simulink model "Model"  (Simulink 7.1)
settings: Solver=ode3  StartTime=0.0  StopTime=30.0  FixedStep=0.01  RelTol=1e-3
settings Model: Creator=Michal  LastModifiedBy=Michal

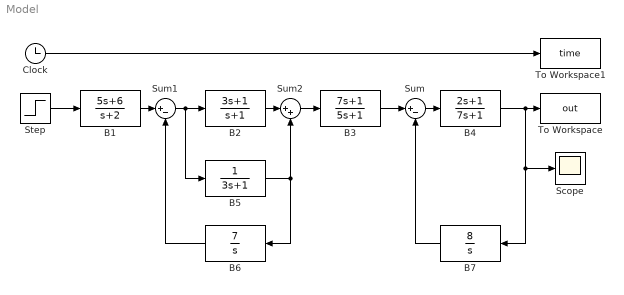
== system Model ==
  B1 : TransferFcn  Numerator=[5 6 ]  Denominator=[1 2]
  B2 : TransferFcn  Numerator=[3 1]  Denominator=[1 1]
  B3 : TransferFcn  Numerator=[7 1]  Denominator=[5 1]
  B4 : TransferFcn  Numerator=[2 1]  Denominator=[7 1]
  B5 : TransferFcn  Denominator=[3 1]
  B6 : TransferFcn  Orientation=left  Numerator=[7]  Denominator=[1 0]
  B7 : TransferFcn  Orientation=left  Numerator=[8]  Denominator=[1 0]
  Clock : Clock
      settings: Decimation=10
  Scope : Scope
      settings: TimeRange=30
  Step : Step  Time=0  SampleTime=0
  Sum : Sum  Inputs=|+-  OutDataType=sfix(16)  OutScaling=2^0
  Sum1 : Sum  Inputs=|+-  OutDataType=sfix(16)  OutScaling=2^0
  Sum2 : Sum  Inputs=|++  OutDataType=sfix(16)  OutScaling=2^0
  To Workspace : ToWorkspace  VariableName=out  SampleTime=-1  SaveFormat=Array
  To Workspace1 : ToWorkspace  VariableName=time  SampleTime=-1  SaveFormat=Array
  wires:
  Step/1 -> B1/1
  B4/1 -> To Workspace/1, B7/1, Scope/1
  B1/1 -> Sum1/1
  Sum1/1 -> B5/1, B2/1
  B6/1 -> Sum1/2
  B2/1 -> Sum2/1
  B5/1 -> Sum2/2, B6/1
  Sum2/1 -> B3/1
  B3/1 -> Sum/1
  Sum/1 -> B4/1
  B7/1 -> Sum/2
  Clock/1 -> To Workspace1/1
